simulink model "LMI_lema_8_statefeedback"  (Simulink 7.7)
settings: Solver=ode45  StartTime=0.0  StopTime=1900  RelTol=1e-3
values from neighbouring files (symbols this model uses):
  QT =     [FaseMinima.mat]    (also in FaseNaoMinima.mat; FaseNaoMinimaMudandoApenasGama.mat; settup.m = dynamics())
settings Model: Creator=Arthur  LastModifiedBy=Arthur
settings DebuggingCC: UnderspecifiedInitializationDetection=Simplified

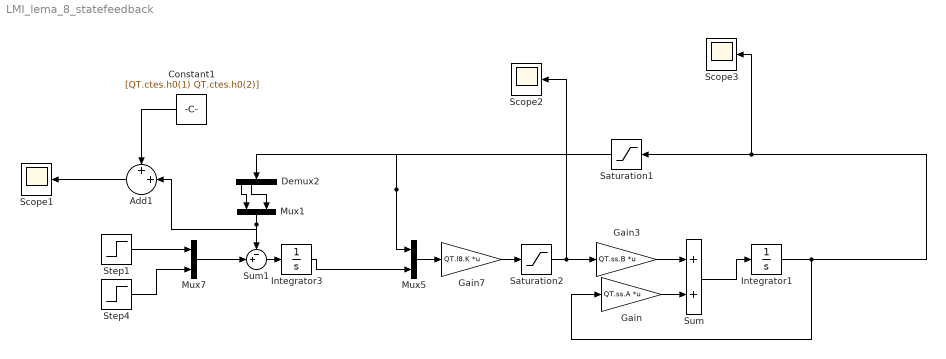
== system LMI_lema_8_statefeedback ==
  Add1 : Sum  Inputs=++|
  Constant1 : Constant  Value=[QT.ctes.h0(1) QT.ctes.h0(2)]
  Demux2 : Demux
  Gain : Gain  Gain=QT.ss.A  Multiplication=Matrix(K*u)
  Gain3 : Gain  Gain=QT.ss.B  Multiplication=Matrix(K*u)
  Gain7 : Gain  Gain=QT.l8.K  Multiplication=Matrix(K*u)
  Integrator1 : Integrator
  Integrator3 : Integrator
  Mux1 : Mux  Inputs=2
  Mux5 : Mux  Inputs=2
  Mux7 : Mux  Inputs=2
  Saturation1 : Saturate  UpperLimit=10  LowerLimit=-10
  Saturation2 : Saturate  UpperLimit=+1.5  LowerLimit=-1.5
  Scope1 : Scope
      settings: TimeRange=10  SaveName=Simulado
  Scope2 : Scope
      settings: TimeRange=100  YMin=-1.1  YMax=0.2  SampleTime=1
  Scope3 : Scope
      settings: TimeRange=100  YMin=0  YMax=1  SaveName=ScopeData2  SampleTime=1
  Step1 : Step  Time=300  SampleTime=0
  Step4 : Step  Time=1100  SampleTime=0
  Sum : Sum
  Sum1 : Sum  Inputs=-+|
  wires:
  Gain/1 -> Sum/2
  Gain3/1 -> Sum/1
  Integrator1/1 -> Gain/1, Scope3/1, Saturation1/1
  Sum/1 -> Integrator1/1
  Gain7/1 -> Saturation2/1
  Mux5/1 -> Gain7/1
  Integrator3/1 -> Mux5/2
  Sum1/1 -> Integrator3/1
  Demux2/1 -> Mux1/1
  Demux2/2 -> Mux1/2
  Mux1/1 -> Sum1/1, Add1/2
  Saturation1/1 -> Mux5/1, Demux2/1
  Saturation2/1 -> Gain3/1, Scope2/1
  Step1/1 -> Mux7/1
  Step4/1 -> Mux7/2
  Mux7/1 -> Sum1/2
  Add1/1 -> Scope1/1
  Constant1/1 -> Add1/1
